simulink model "DCAC_conv_intconv_VSM"  (R2025a)
settings: Solver=VariableStepAuto  StartTime=0.0  StopTime=10.0  RelTol=1e-3
undefined symbols (not defined in the file): fb, Grid_op_VCVSC, Grid_op_VSM, Grid_opDC_VSM, Grid_opintconv_VSM, Grid_opVCVSC
libraries: simulink x1
(part 1 of 2)
settings Model: Creator=atomas  LastModifiedBy=atomas

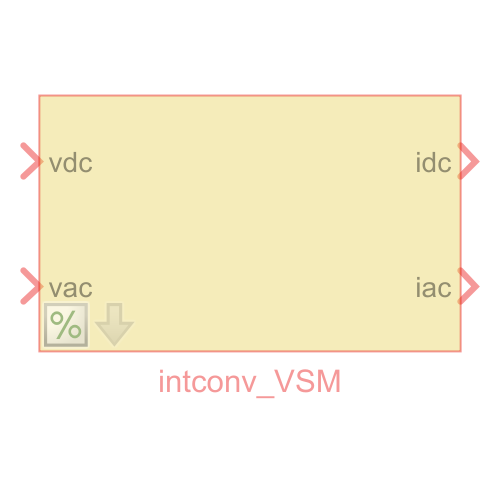
[thumbnail: Simulink's stored preview of the top-level diagram]
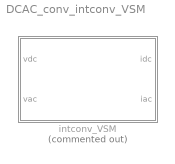
== system DCAC_conv_intconv_VSM ==
  intconv_VSM : Subsystem  Commented=on  mask(VCVSC){dynamic_VCC=Dynamic with P limitation, Lf=0.1, Rf=0.01, Rcf=1000000, Cfi=0.1, Kint=1, Tint=0.1, Bint=1, Kext=1, Bext=1, Text=0.1, Fi=1, Hv=3, Dv=0, Rv=0.05, nq=0.05, VI_L=0, VI_R=0, WOF_Tf=0, L_out=0.1, R_out=0.01}
      mask prompts: dynamic_VCC "Dynamic behavior"; Lf "Filter inductance (pu)"; Rf "Filter resistance (pu)"; Rcf "Parallel resistance to C (pu)"; Cfi "Filter capacitance (pu)"; Fi "Current feedfordward gain"; Hv "Inertia"; Dv "Damping"; Rv "Droop Rv"; nq "Droop nq"; VI_L "Inductance (pu)"; VI_R "Resistance (pu)"; WOF_Tf "WOF time constant (s)"; L_out "Output inductance (p.u.)"; R_out "Output resistance (p.u.)"
      mask help: Grid-forming converter. VCC are the voltage and current controllers. Dynamic behavior includes the PI controllers, decoupling, current feedfordward and LC output filter. Static behavior consists of setting the reference voltage directly in the output. PC is the power controller including the droop control and low-pass filters for the power measurements.
      mask init:
      | mdlWks = get_param(bdroot,'ModelWorkspace'); % Get the model workspace
      | block_name = get_param(gcb,'Name');
      | bvarname = get_param(get_param(get_param(...
      |         gcb, 'Parent'), 'Parent'), 'bvarname');
      | DC = mdlWks.getVariable([bvarname 'DC']);
      | try
      |     block_DC_buses = DC.(block_name + "s_DC_buses");
      |     block_buses = DC.(block_name + "s_buses");
      |     block_DC_toM = DC.(block_name + "s_DC_toM");
      |     block_toM = DC.(block_name + "s_toM");
      |     dparams = DC.(block_name + "_dparams");
      |     fref = mdlWks.getVariable([bvarname 'fref']);
      |     block_fref = fref.(block_name);
      | catch ME
      |     %errordlg(ME.message) 
      | end
      mask Help: web('Documentation/VCVSC.html')
      mask TypeOptions dynamic_VCC: Dynamic with limitation | Dynamic with P limitation | Dynamic | Static | Dynamic VC and static CC
      mask Callback dynamic_VCC:
      | block = gcb;
      | dynamic = get_param(block, 'dynamic_VCC');
      | param_vis = get_param(block,'MaskVisibilities');
      | block_params = string(fieldnames(get_param(block, 'DialogParameters')));
      | switch dynamic
      |     case 'Dynamic'
      |         param_vis(find(block_params == 'Lf'):find(block_params == 'Fi')) = cellstr("on");
      |         set_param([gcb '/VCC'], 'LabelModeActiveChoice', 'dynamic');
      |     case 'Dynamic with limitation'
      |         param_vis(find(block_params == 'Lf'):find(block_params == 'Fi')) = cellstr("on");
      |         set_param([gcb '/VCC'], 'LabelModeActiveChoice', 'dynamic_limiting');
      |     case 'Dynamic with P limitation'
      |         param_vis(find(block_params == 'Lf'):find(block_params == 'Fi')) = cellstr("on");
      |         set_param([gcb '/VCC'], 'LabelModeActiveChoice', 'dynamic_limiting_P');
      |     case 'Static'
      |         param_vis(find(block_params == 'Lf'):find(block_params == 'Fi')) = cellstr("off");
      |         set_param([gcb '/VCC'], 'LabelModeActiveChoice', 'static');
      |     case 'Dynamic VC and static CC'
      |         param_vis(find(block_params == 'Lf'):find(block_params == 'Fi')) = cellstr("on");
      |         param_vis(ismember(block_params, ["Lf","Rf","Kpc","Kic","Fi"])) = cellstr("off");
      |         set_param([gcb '/VCC'], 'LabelModeActiveChoice', 'dynamic_VC');
      | end
      | set_param(block,'MaskVisibilities',param_vis)
      mask TypeOptions VI_L: VI/L
      mask TypeOptions VI_R: VI/R
      mask TypeOptions WOF_Tf: VI/Tf
      mask DialogControl Container8 Prompt: Parameters
      mask DialogControl VCC Prompt: VCC
      mask DialogControl PC Prompt: PC
      mask DialogControl VI Prompt: VI
      mask DialogControl Container9 Prompt: Others

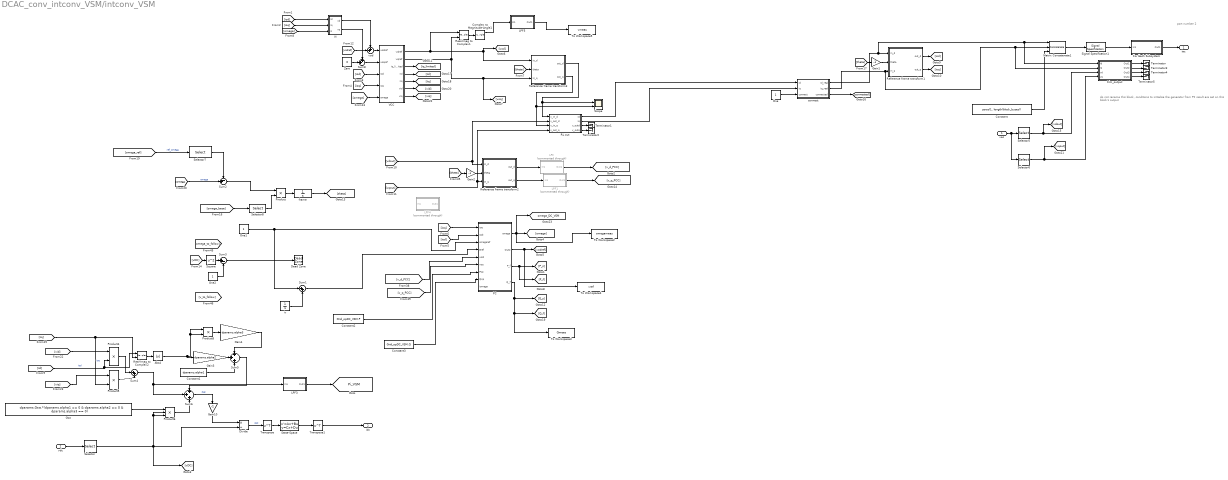
== system DCAC_conv_intconv_VSM/intconv_VSM ==
  note: port number 2
  note: do not rename this block, conditions to initialise the generator from PF result are set on this block's output
  vac : Inport
  vdc : Inport  Port=2
  Abs4 : Abs  SaturateOnIntegerOverflow=off
  Complex to Magnitude-Angle1 : ComplexToMagnitudeAngle
  Constant : Constant  Value=zeros(1, length(block_buses))  VectorParams1D=off
  Constant1 : Constant  Value=dparams.alpha1  VectorParams1D=off
  Constant2 : Constant  Value=Grid_opDC_VSM.P
  Constant3 : Constant  Value=Grid_opDC_VSM.Q
  Dead Zone : DeadZone  LowerValue=-0.2  UpperValue=0.2
  Divide : Product  Inputs=*/
  For Each Subsystem : Subsystem  TreatAsAtomicUnit=on
  Gain1 : Gain  Gain=-1
  Gain10 : Gain  Gain=-1
  Gain2 : Gain  Gain=-1
  Gain3 : Gain  Gain=dparams.alpha2
  Gain4 : Gain  Gain=dparams.alpha3
  Gsw : Constant  Value=dparams.Gsw.*(dparams.alpha1 == 0 & dparams.alpha2 == 0 & dparams.alpha3 == 0)  VectorParams1D=off
  LPF : Subsystem  Commented=through
  LPF1 : Subsystem  Commented=through
  LPF3 : Subsystem
  LPF4 : Subsystem  Commented=through
  LPF5 : Subsystem
  Matrix Concatenate1 : Concatenate  NumInputs=3  Mode=Multidimensional array
  One : Constant  OutDataTypeStr=Inherit: Inherit via back propagation
  One1 : Constant  OutDataTypeStr=Inherit: Inherit via back propagation
  One2 : Constant  OutDataTypeStr=Inherit: Inherit via back propagation
  PC : Subsystem  mask(PC_VCVSC){Tf=0.01, mp=0.01, nq=nq}
      mask prompts: Tf "Low-pass filter time constant (s)"; mp "Droop coefficient mp"; nq "Droop coefficient nq"
      mask help: Power controller of a grid-forming converter, including the droop control and low-pass filters for the power measurements.
      mask init:
      | if all(Tf ~= 0)
      |     iTf = 1./Tf;
      |     set_param([gcb '/LPF_P'],'Commented','off')
      |     set_param([gcb '/LPF_Q'],'Commented','off')
      | else
      |     set_param([gcb '/LPF_P'],'Commented','through')
      |     set_param([gcb '/LPF_Q'],'Commented','through')
      | end
  Product{,4..5,8} (4 alike) : Product
  Product6 : Product  Inputs=3
  RL out : Subsystem  Variant=on  VariantControlMode=label  LabelModeActiveChoice=dynamic  mask{dynamic=Dynamic, R=dparams.Rf, L=dparams.Lf, fbase=50}
      mask prompts: dynamic "Dynamic behavior"; R "Series resistance (p.u.)"; L "Inductance (p.u.)"; fbase "Base frequency (Hz)"
      mask init:
      | omegab = 2*pi*fbase;
      | invL = 1./L;
      | vssBlk = gcb;
      | switch dynamic
      |     case "Static"
      |         set_param(vssBlk, 'LabelModeActiveChoice', 'static');
      |     case "Dynamic"
      |         set_param(vssBlk, 'LabelModeActiveChoice', 'dynamic');
      |     case "Static omega"
      |         set_param(vssBlk, 'LabelModeActiveChoice', 'static_omega');
      | end
      mask TypeOptions dynamic: Static | Dynamic | Static omega
  Real-Imag to Complex1 : RealImagToComplex
  Real-Imag to Complex2 : RealImagToComplex
  Reference frame transform1 : Subsystem
  Reference frame transform2 : Subsystem
  Reference frame transform3 : Subsystem
  Scope : Scope  NumInputPorts=2
      settings: ActiveDisplayYMinimum=0.95813  ActiveDisplayYMaximum=1.0211
  Selector : Selector  InputPortWidth=DC.Nbuses  IndexOptions=Index vector (dialog)  Indices=block_DC_buses  OutputSizes=1
  Selector5 : Selector  NumberOfDimensions=2  InputPortWidth=3  IndexOptions=Index vector (dialog),Index vector (dialog)  Indices=1,block_buses  OutputSizes=1,1
  Selector6 : Selector  NumberOfDimensions=2  InputPortWidth=3  IndexOptions=Index vector (dialog),Index vector (dialog)  Indices=2,block_buses  OutputSizes=1,1
  Selector7 : Selector  InputPortWidth=length(fref.ref_units)  IndexOptions=Index vector (dialog)  Indices=block_fref  OutputSizes=1
  Selector8 : Selector  InputPortWidth=length(fref.ref_units)  IndexOptions=Index vector (dialog)  Indices=block_fref  OutputSizes=1
  Signal Specification1 : SignalSpecification  Dimensions=[3 length(block_buses)]
  Square : Math  Operator=square
  State-Space : StateSpace  A=[]  B=[]  C=[]  D=block_DC_toM  InitialCondition=0  ParameterTunability=Optimized
  Sum1 : Sum  Inputs=|++
  Sum2 : Sum  Inputs=-+|
  Sum3 : Sum  Inputs=|+-
  Sum4 : Sum  Inputs=|++
  Sum5 : Sum  Inputs=+|+|+
  Sum6 : Sum  Inputs=+|+|+
  Sum8 : Sum  Inputs=++|
  Terminator{,1..5} (6 alike) : Terminator
  To Workspace2 : ToWorkspace  VariableName=omegameas  SaveFormat=Timeseries  SampleTime=-1
  To Workspace3 : ToWorkspace  VariableName=Qmeas  SaveFormat=Timeseries  SampleTime=-1
  To Workspace4 : ToWorkspace  VariableName=vref  SaveFormat=Timeseries  SampleTime=-1
  To Workspace5 : ToWorkspace  VariableName=vmeas  SaveFormat=Timeseries  SampleTime=-1
  Transpose : Math  Operator=transpose
  Transpose1 : Math  Operator=transpose
  VCC : Subsystem  Variant=on  VariantControlMode=label  LabelModeActiveChoice=dynamic_limiting_P
  VI : Subsystem  mask{L=VI_L, R=VI_R, Tf=WOF_Tf}
      mask prompts: L "Inductance (pu)"; R "Resistance (pu)"; Tf "WOF time constant (s)"
      mask init:
      | if all(Tf ~= 0)
      |     iTf = 1./Tf;
      |     set_param([gcb '/WOF_d'],'Commented','off')
      |     set_param([gcb '/WOF_q'],'Commented','off')
      | else
      |     set_param([gcb '/WOF_d'],'Commented','through')
      |     set_param([gcb '/WOF_q'],'Commented','through')
      | end
  Zero : Constant  Value=0  OutDataTypeStr=Inherit: Inherit via back propagation
  connect : Subsystem
  frame : Integrator  InitialCondition=Grid_opintconv_VSM.frame  IgnoreLimit=on
  iv : Integrator  InitialCondition=Grid_opintconv_VSM.iv
  trim_output : Subsystem
  vod : Sum  Inputs=++|
  iac : Outport
  idc : Outport  Port=2
  tag scope: Pi_VSM=global, omega_DC_VSM=global
  wires:
  Selector7/1 -> Sum2/1
  Sum2/1 -> Product/1
  [omega_base] -> Selector8/1
  Selector8/1 -> Product/2
  LPF5/1(Out1) -> To Workspace5/1
  Complex to Magnitude-Angle1/1 -> LPF5/1(In1)
  Real-Imag to Complex1/1 -> Complex to Magnitude-Angle1/1
  LPF3/1(Out1) -> [Pi_VSM]
  Sum3/1 -> Dead Zone/1
  frame/1 -> [theta]
  One2/1 -> Sum3/2
  Square/1 -> Sum3/1
  [vDC] -> Square/1
  One1/1 -> Sum1/1, PC/3(omegaref)
  VCC/7(viq) -> [viq]
  VCC/6(vid) -> [vid]
  VCC/5(iiq) -> [iiq]
  VCC/4(iid) -> [iid]
  VCC/3(iq_limited) -> [iq_limited]
  Product/1 -> frame/1
  [iid] -> Real-Imag to Complex2/1, Product4/2  "iod"
  [vid] -> Product4/1
  [iiq] -> Real-Imag to Complex2/2, Product5/2  "ioq"
  Selector/1 -> Divide/2, [vDC], Product6/2, Product6/3
  [viq] -> Product5/1
  Product8/1 -> Gain4/1
  Gain10/1 -> Divide/1
  Gain3/1 -> Sum5/2
  Sum6/1 -> Gain10/1  "Pdc"
  Product4/1 -> Sum4/1
  Constant1/1 -> Sum5/3
  Real-Imag to Complex2/1 -> Abs4/1
  Gsw/1 -> Product6/1
  Gain4/1 -> Sum5/1
  State-Space/1 -> Transpose1/1
  Sum5/1 -> Sum6/1
  Sum4/1 -> Sum6/2, LPF3/1(In1)
  Product6/1 -> Sum6/3
  Product5/1 -> Sum4/2
  Transpose1/1 -> idc/1
  Abs4/1 -> Gain3/1, Product8/1, Product8/2
  Divide/1 -> Transpose/1  "iDC"
  Transpose/1 -> State-Space/1
  vdc/1 -> Selector/1
  Sum1/1 -> PC/4(Eref)
  One/1 -> connect/3(connect)
  iv/1 -> Sum1/2
  Constant3/1 -> PC/8(Qsp)
  Constant2/1 -> PC/7(Psp)
  VCC/2(viqref) -> Real-Imag to Complex1/2, Reference frame transform3/3(in_q), [voq]
  VCC/1(vidref) -> Reference frame transform3/1(in_d), [vod], Real-Imag to Complex1/1
  Selector5/1 -> trim_output/3(vd), [vdout]
  Selector6/1 -> trim_output/4(vq), [vqout]
  vac/1 -> Selector5/1, Selector6/1
  trim_output/4(Out4) -> Terminator5/1
  trim_output/3(Out3) -> Terminator4/1
  trim_output/2(Out2) -> Terminator3/1
  trim_output/1(Out1) -> Terminator/1
  [v_q_PCC] -> PC/6(voq)
  [v_d_PCC] -> PC/5(vodi)
  Signal Specification1/1 -> For Each Subsystem/1(In1)
  For Each Subsystem/1(Out1) -> iac/1
  Constant/1 -> Matrix Concatenate1/3
  Matrix Concatenate1/1 -> Signal Specification1/1
  [vdout] -> Reference frame transform2/1(in_d), RL out/2(v_out_d)
  LPF1/1(Out1) -> [v_q_PCC]
  LPF/1(Out1) -> [v_d_PCC]
  [vqout] -> RL out/4(v_out_q), Reference frame transform2/3(in_q)
  Reference frame transform2/2(out_q) -> LPF1/1(In1)
  Reference frame transform2/1(out_d) -> LPF/1(In1)
  RL out/4(v_outq) -> Terminator2/1
  RL out/3(v_outd) -> Terminator1/1
  connect/2(iq_real) -> Reference frame transform1/3(in_q), Matrix Concatenate1/2, trim_output/2(iq)
  connect/1(id_real) -> Reference frame transform1/1(in_d), Matrix Concatenate1/1, trim_output/1(id)
  VI/2(vq) -> Sum8/1
  VI/1(vd) -> vod/1
  Reference frame transform1/1(out_d) -> [iod]
  RL out/2(iq) -> connect/2(iq)
  Reference frame transform3/2(out_q) -> Scope/2, RL out/3(v_in_q)
  Reference frame transform3/1(out_d) -> Scope/1, RL out/1(v_in_d)
  Reference frame transform1/2(out_q) -> [ioq]
  [ioq] -> PC/1(ioq)
  [iod] -> PC/2(iodi)
  PC/2(Out2) -> [vodref], To Workspace4/1
  PC/1(omega) -> [omega], [omega_DC_VSM], To Workspace2/1
  [theta] -> Reference frame transform3/2(theta)
  [omega] -> VCC/5(omega)
  [vodref] -> vod/2
  Zero/1 -> Sum8/2
  [iod] -> VCC/3(iod)
  [ioq] -> VCC/4(ioq)
  Gain1/1 -> Reference frame transform1/2(theta)
  [theta] -> Gain1/1
  RL out/1(id) -> connect/1(id)
  [omega_ref] -> Selector7/1  "ref_omega"
  [omega] -> Sum2/2  "omega"
  connect/3(connected) -> [connected]
  PC/3(P_f) -> [P_f], [P_s]
  PC/4(Q_f) -> [Q_f], To Workspace3/1, [Q_s]
  [theta] -> Gain2/1
  Gain2/1 -> Reference frame transform2/2(theta)
  [iod] -> VI/1(id)
  [ioq] -> VI/2(iq)
  [omega] -> VI/3(omega)
  vod/1 -> VCC/1(vodref)
  Sum8/1 -> VCC/2(voqref)

== system DCAC_conv_intconv_VSM/intconv_VSM/For Each Subsystem ==
  In1 : Inport  Partition=on  PartitionDimension=1  PartitionWidth=1  PartitionOffset=0
  For Each : ForEach  DisableCoverage=on
  State-Space : StateSpace  A=[]  B=[]  C=[]  D=block_toM  InitialCondition=0  ParameterTunability=Optimized
  Transpose : Math  Operator=transpose
  Transpose1 : Math  Operator=transpose
  Out1 : Outport  ConcatenationDimension=1
  wires:
  In1/1 -> Transpose/1
  Transpose1/1 -> Out1/1
  Transpose/1 -> State-Space/1
  State-Space/1 -> Transpose1/1

== system DCAC_conv_intconv_VSM/intconv_VSM/LPF ==
  In1 : Inport
  Gain : Gain  Gain=1e2
  I : Integrator  InitialCondition=Grid_op_VCVSC.op.States(4).x'
  Sum4 : Sum  Inputs=|+-
  Out1 : Outport
  wires:
  I/1 -> Sum4/2, Out1/1
  In1/1 -> Sum4/1
  Sum4/1 -> Gain/1
  Gain/1 -> I/1

== system DCAC_conv_intconv_VSM/intconv_VSM/LPF1 ==
  In1 : Inport
  Gain : Gain  Gain=1e2
  I : Integrator  InitialCondition=Grid_op_VCVSC.op.States(5).x'
  Sum4 : Sum  Inputs=|+-
  Out1 : Outport
  wires:
  Gain/1 -> I/1
  Sum4/1 -> Gain/1
  In1/1 -> Sum4/1
  I/1 -> Out1/1, Sum4/2

== system DCAC_conv_intconv_VSM/intconv_VSM/LPF3 ==
  In1 : Inport
  Gain : Gain  Gain=1000
  I : Integrator
  Sum4 : Sum  Inputs=|+-
  Out1 : Outport
  wires:
  I/1 -> Sum4/2, Out1/1
  In1/1 -> Sum4/1
  Sum4/1 -> Gain/1
  Gain/1 -> I/1

== system DCAC_conv_intconv_VSM/intconv_VSM/LPF4 ==
  In1 : Inport
  Gain : Gain  Gain=1e2
  I : Integrator
  Sum4 : Sum  Inputs=|+-
  Out1 : Outport
  wires:
  I/1 -> Sum4/2, Out1/1
  In1/1 -> Sum4/1
  Sum4/1 -> Gain/1
  Gain/1 -> I/1

== system DCAC_conv_intconv_VSM/intconv_VSM/LPF5 ==
  In1 : Inport
  Gain : Gain  Gain=1e4
  I : Integrator  InitialConditionSource=external
  Sum4 : Sum  Inputs=|+-
  Out1 : Outport
  wires:
  I/1 -> Sum4/2, Out1/1
  In1/1 -> Sum4/1, I/2
  Sum4/1 -> Gain/1
  Gain/1 -> I/1

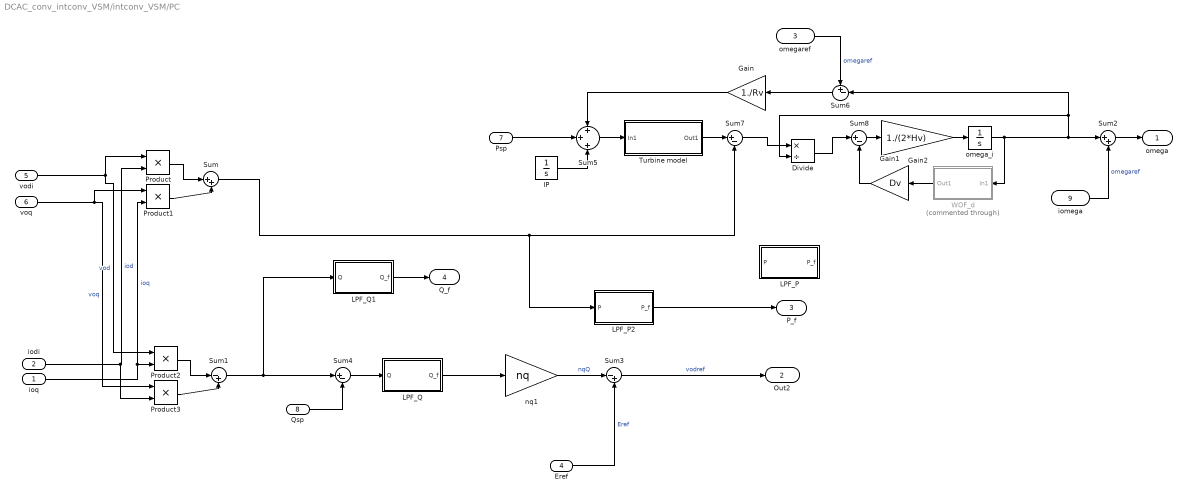
== system DCAC_conv_intconv_VSM/intconv_VSM/PC ==
  ioq : Inport
  iodi : Inport  Port=2
  omegaref : Inport  Port=3
  Eref : Inport  Port=4
  vodi : Inport  Port=5
  voq : Inport  Port=6
  Psp : Inport  Port=7
  Qsp : Inport  Port=8
  iomega : Inport  Port=9
  Divide : Product  Inputs=*/
  Gain : Gain  Gain=1./Rv
  Gain1 : Gain  Gain=Dv
  Gain2 : Gain  Gain=1./(2*Hv)
  IP : Integrator  InitialCondition=Grid_opintconv_VSM.IP
  LPF_P : Subsystem
  LPF_P2 : Subsystem
  LPF_Q : Subsystem
  LPF_Q1 : Subsystem
  Product{,1..3} (4 alike) : Product
  Sum : Sum  Inputs=|++
  Sum1 : Sum  Inputs=|-+
  Sum2 : Sum  Inputs=|++
  Sum3 : Sum  Inputs=|-+
  Sum4 : Sum  Inputs=|+-
  Sum5 : Sum  Inputs=+|+|+
  Sum6 : Sum  Inputs=+-|
  Sum7 : Sum  Inputs=|+-
  Sum8 : Sum  Inputs=|+-
  Turbine model : Subsystem
  WOF_d : Subsystem  Commented=through
  nq1 : Gain  Gain=nq
  omega_i : Integrator  InitialCondition=1
  omega : Outport
  Out2 : Outport  Port=2
  P_f : Outport  Port=3
  Q_f : Outport  Port=4
  wires:
  LPF_Q1/1(Q_f) -> Q_f/1
  LPF_P2/1(P_f) -> P_f/1
  iomega/1 -> Sum2/2  "omegaref"
  Sum2/1 -> omega/1
  omegaref/1 -> Sum6/1  "omegaref"
  IP/1 -> Sum5/3
  Sum8/1 -> Gain2/1
  Sum7/1 -> Divide/1
  Sum5/1 -> Turbine model/1(In1)
  Psp/1 -> Sum5/2
  Divide/1 -> Sum8/1
  Gain1/1 -> Sum8/2
  Turbine model/1(Out1) -> Sum7/1
  WOF_d/1(Out1) -> Gain1/1
  Gain/1 -> Sum5/1
  omega_i/1 -> Divide/2, Sum6/2, Sum2/1, WOF_d/1(In1)
  Sum/1 -> LPF_P2/1(P), Sum7/2
  Sum6/1 -> Gain/1
  Gain2/1 -> omega_i/1
  LPF_Q/1(Q_f) -> nq1/1
  Sum3/1 -> Out2/1  "vodref"
  Sum4/1 -> LPF_Q/1(Q)
  Qsp/1 -> Sum4/2
  ioq/1 -> Product1/2, Product2/2  "ioq"
  iodi/1 -> Product/2, Product3/2  "iod"
  voq/1 -> Product3/1, Product1/1  "voq"
  Sum1/1 -> Sum4/1, LPF_Q1/1(Q)
  Eref/1 -> Sum3/2  "Eref"
  nq1/1 -> Sum3/1  "nqQ"
  Product3/1 -> Sum1/2
  Product2/1 -> Sum1/1
  Product1/1 -> Sum/2
  Product/1 -> Sum/1
  vodi/1 -> Product/1, Product2/1  "vod"

== system DCAC_conv_intconv_VSM/intconv_VSM/RL out ==
  note: 1) Add Subsystem or Model blocks as valid variant choices.
      | 2) You cannot connect blocks at this level. At simulation, connectivity is automatically
      | determined, based on the active variant and port name matching.
  v_in_d : Inport
  v_out_d : Inport  Port=2
  v_in_q : Inport  Port=3
  v_out_q : Inport  Port=4
  dynamic : Subsystem  VariantControl=dynamic
  static : Subsystem  VariantControl=static
  static_omega : Subsystem  VariantControl=static_omega
  id : Outport
  iq : Outport  Port=2
  v_outd : Outport  Port=3
  v_outq : Outport  Port=4

== system DCAC_conv_intconv_VSM/intconv_VSM/Reference frame transform1 ==
  in_d : Inport
  theta : Inport  Port=2
  in_q : Inport  Port=3
  Complex to Real-Imag : ComplexToRealImag
  Cos : Trigonometry  SCDEnableBlockLinearizationSpecification=on  Operator=cos
  Product : Product
  Real-Imag to Complex : RealImagToComplex
  Real-Imag to Complex1 : RealImagToComplex
  Sin : Trigonometry  SCDEnableBlockLinearizationSpecification=on
  out_d : Outport
  out_q : Outport  Port=2
  wires:
  in_d/1 -> Real-Imag to Complex/1
  in_q/1 -> Real-Imag to Complex/2
  Complex to Real-Imag/1 -> out_d/1
  Sin/1 -> Real-Imag to Complex1/2
  Cos/1 -> Real-Imag to Complex1/1
  theta/1 -> Cos/1, Sin/1
  Product/1 -> Complex to Real-Imag/1
  Real-Imag to Complex/1 -> Product/2
  Real-Imag to Complex1/1 -> Product/1
  Complex to Real-Imag/2 -> out_q/1

== system DCAC_conv_intconv_VSM/intconv_VSM/Reference frame transform2 ==
  in_d : Inport
  theta : Inport  Port=2
  in_q : Inport  Port=3
  Complex to Real-Imag : ComplexToRealImag
  Cos : Trigonometry  SCDEnableBlockLinearizationSpecification=on  Operator=cos
  Product : Product
  Real-Imag to Complex : RealImagToComplex
  Real-Imag to Complex1 : RealImagToComplex
  Sin : Trigonometry  SCDEnableBlockLinearizationSpecification=on
  out_d : Outport
  out_q : Outport  Port=2
  wires:
  Complex to Real-Imag/2 -> out_q/1
  Real-Imag to Complex1/1 -> Product/1
  Real-Imag to Complex/1 -> Product/2
  Product/1 -> Complex to Real-Imag/1
  theta/1 -> Sin/1, Cos/1
  Cos/1 -> Real-Imag to Complex1/1
  Sin/1 -> Real-Imag to Complex1/2
  Complex to Real-Imag/1 -> out_d/1
  in_q/1 -> Real-Imag to Complex/2
  in_d/1 -> Real-Imag to Complex/1

== system DCAC_conv_intconv_VSM/intconv_VSM/Reference frame transform3 ==
  in_d : Inport
  theta : Inport  Port=2
  in_q : Inport  Port=3
  Complex to Real-Imag : ComplexToRealImag
  Cos : Trigonometry  SCDEnableBlockLinearizationSpecification=on  Operator=cos
  Product : Product
  Real-Imag to Complex : RealImagToComplex
  Real-Imag to Complex1 : RealImagToComplex
  Sin : Trigonometry  SCDEnableBlockLinearizationSpecification=on
  out_d : Outport
  out_q : Outport  Port=2
  wires:
  in_d/1 -> Real-Imag to Complex/1
  in_q/1 -> Real-Imag to Complex/2
  Complex to Real-Imag/1 -> out_d/1
  Sin/1 -> Real-Imag to Complex1/2
  Cos/1 -> Real-Imag to Complex1/1
  theta/1 -> Sin/1, Cos/1
  Product/1 -> Complex to Real-Imag/1
  Real-Imag to Complex/1 -> Product/2
  Real-Imag to Complex1/1 -> Product/1
  Complex to Real-Imag/2 -> out_q/1

== system DCAC_conv_intconv_VSM/intconv_VSM/VCC ==
  note: 1) Add Subsystem or Model blocks as valid variant choices.
      | 2) You cannot connect blocks at this level. At simulation, connectivity is automatically
      | determined, based on the active variant and port name matching.
  vodref : Inport
  voqref : Inport  Port=2
  iod : Inport  Port=3
  ioq : Inport  Port=4
  omega : Inport  Port=5
  dynamic : Subsystem  VariantControl=dynamic
  dynamic_VC : Subsystem  VariantControl=dynamic_VC
  dynamic_limiting : Subsystem  VariantControl=dynamic_limiting
  dynamic_limiting_P : Subsystem  VariantControl=dynamic_limiting_P
  static : Subsystem  VariantControl=static
  vidref : Outport
  viqref : Outport  Port=2
  iq_limited : Outport  Port=3
  iid : Outport  Port=4
  iiq : Outport  Port=5
  vid : Outport  Port=6
  viq : Outport  Port=7

== system DCAC_conv_intconv_VSM/intconv_VSM/VI ==
  id : Inport
  iq : Inport  Port=2
  omega : Inport  Port=3
  Gain : Gain  Gain=L
  Gain1 : Gain  Gain=R
  Gain2 : Gain  Gain=L
  Gain3 : Gain  Gain=R
  Product : Product
  Product1 : Product
  Sum : Sum  Inputs=-+|
  Sum1 : Sum  Inputs=|--
  WOF_d : Subsystem  Commented=through
  WOF_q : Subsystem  Commented=through
  vd : Outport
  vq : Outport  Port=2
  wires:
  Gain/1 -> Product/1
  omega/1 -> Product/2, Product1/1
  iq/1 -> WOF_q/1(In1)
  Product/1 -> Sum/2
  id/1 -> WOF_d/1(In1)
  Gain2/1 -> Product1/2
  Product1/1 -> Sum1/1
  Gain1/1 -> Sum/1
  Gain3/1 -> Sum1/2
  Sum/1 -> vd/1
  Sum1/1 -> vq/1
  WOF_d/1(Out1) -> Gain2/1, Gain1/1
  WOF_q/1(Out1) -> Gain3/1, Gain/1

== system DCAC_conv_intconv_VSM/intconv_VSM/connect ==
  id : Inport
  iq : Inport  Port=2
  connect : Inport  Port=3
  Switch : Switch  Criteria=u2 > Threshold  ZeroCross=off  SaturateOnIntegerOverflow=off  InputSameDT=off
  Switch1 : Switch  Criteria=u2 > Threshold  ZeroCross=off  SaturateOnIntegerOverflow=off  InputSameDT=off
  Zero1 : Constant  Value=0  VectorParams1D=off  OutDataTypeStr=Inherit: Inherit via back propagation
  Zero2 : Constant  Value=0  VectorParams1D=off  OutDataTypeStr=Inherit: Inherit via back propagation
  id_real : Outport
  iq_real : Outport  Port=2
  connected : Outport  Port=3  OutDataTypeStr=boolean
  wires:
  Zero2/1 -> Switch1/3
  iq/1 -> Switch1/1
  Switch1/1 -> iq_real/1
  connect/1 -> Switch/2, Switch1/2, connected/1
  id/1 -> Switch/1
  Zero1/1 -> Switch/3
  Switch/1 -> id_real/1

== system DCAC_conv_intconv_VSM/intconv_VSM/trim_output ==
  id : Inport
  iq : Inport  Port=2
  vd : Inport  Port=3
  vq : Inport  Port=4
  Out1 : Outport
  Out2 : Outport  Port=2
  Out3 : Outport  Port=3
  Out4 : Outport  Port=4
  wires:
  iq/1 -> Out2/1
  vd/1 -> Out3/1
  vq/1 -> Out4/1
  id/1 -> Out1/1

== system DCAC_conv_intconv_VSM/intconv_VSM/PC/LPF_P ==
  P : Inport
  Gain : Gain  Gain=1e4
  I : Integrator  InitialCondition=Grid_opintconv_VSM.P
  Sum4 : Sum  Inputs=|+-
  P_f : Outport
  wires:
  I/1 -> Sum4/2, P_f/1
  P/1 -> Sum4/1
  Sum4/1 -> Gain/1
  Gain/1 -> I/1

== system DCAC_conv_intconv_VSM/intconv_VSM/PC/LPF_P2 ==
  P : Inport
  Gain : Gain  Gain=1e4
  I : Integrator  InitialCondition=Grid_opDC_VSM.P
  Sum4 : Sum  Inputs=|+-
  P_f : Outport
  wires:
  Gain/1 -> I/1
  Sum4/1 -> Gain/1
  P/1 -> Sum4/1
  I/1 -> P_f/1, Sum4/2

== system DCAC_conv_intconv_VSM/intconv_VSM/PC/LPF_Q ==
  Q : Inport
  Gain : Gain  Gain=iTf
  I : Integrator
  Sum4 : Sum  Inputs=|+-
  Q_f : Outport
  wires:
  Sum4/1 -> Gain/1
  I/1 -> Sum4/2, Q_f/1
  Q/1 -> Sum4/1
  Gain/1 -> I/1

== system DCAC_conv_intconv_VSM/intconv_VSM/PC/LPF_Q1 ==
  Q : Inport
  Gain : Gain  Gain=iTf
  I : Integrator  InitialConditionSource=external
  Sum4 : Sum  Inputs=|+-
  Q_f : Outport
  wires:
  Gain/1 -> I/1
  Q/1 -> Sum4/1, I/2
  I/1 -> Q_f/1, Sum4/2
  Sum4/1 -> Gain/1

== system DCAC_conv_intconv_VSM/intconv_VSM/PC/Turbine model ==
  In1 : Inport
  Out1 : Outport
  wires:
  In1/1 -> Out1/1

== system DCAC_conv_intconv_VSM/intconv_VSM/PC/WOF_d ==
  In1 : Inport
  Gain : Gain  Gain=10
  Gain1 : Gain  Gain=10
  I : Integrator  InitialConditionSource=external  InitialCondition=Grid_op_VSM.op.States(7).x'
  Sum : Sum  Inputs=+-|
  Sum4 : Sum  Inputs=|+-
  Out1 : Outport
  wires:
  Gain1/1 -> Out1/1
  Sum/1 -> Gain1/1
  I/1 -> Sum4/2, Sum/2
  In1/1 -> Sum4/1, Sum/1, I/2
  Sum4/1 -> Gain/1
  Gain/1 -> I/1

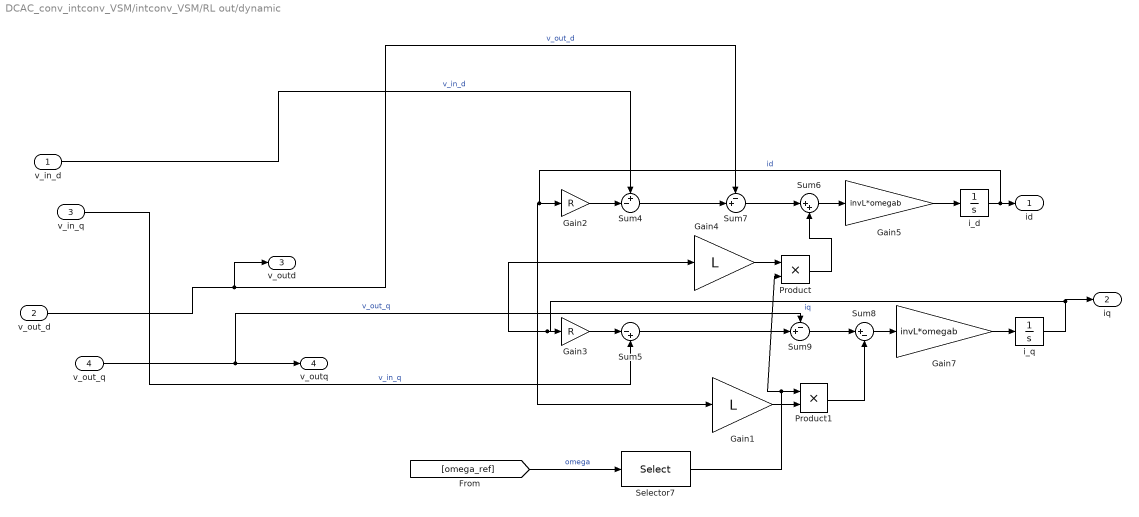
== system DCAC_conv_intconv_VSM/intconv_VSM/RL out/dynamic ==
  v_in_d : Inport
  v_out_d : Inport  Port=2
  v_in_q : Inport  Port=3
  v_out_q : Inport  Port=4
  Gain1 : Gain  Gain=L
  Gain2 : Gain  Gain=R
  Gain3 : Gain  Gain=R
  Gain4 : Gain  Gain=L
  Gain5 : Gain  Gain=invL*omegab
  Gain7 : Gain  Gain=invL*omegab
  Product : Product
  Product1 : Product
  Selector7 : Selector  InputPortWidth=length(fref.ref_units)  IndexOptions=Index vector (dialog)  Indices=block_fref  OutputSizes=1
  Sum4 : Sum  Inputs=+-|
  Sum5 : Sum  Inputs=|-+
  Sum6 : Sum  Inputs=|++
  Sum7 : Sum  Inputs=-+|
  Sum8 : Sum  Inputs=|+-
  Sum9 : Sum  Inputs=-+|
  i_d : Integrator  InitialCondition=Grid_opintconv_VSM.id_out
  i_q : Integrator  InitialCondition=Grid_opintconv_VSM.iq_out
  id : Outport
  iq : Outport  Port=2
  v_outd : Outport  Port=3
  v_outq : Outport  Port=4
  wires:
  Selector7/1 -> Product1/1, Product/2
  v_in_q/1 -> Sum5/2  "v_in_q"
  v_in_d/1 -> Sum4/1  "v_in_d"
  Gain2/1 -> Sum4/2
  i_d/1 -> Gain2/1, Gain1/1, id/1  "id"
  Sum6/1 -> Gain5/1
  [omega_ref] -> Selector7/1  "omega"
  Gain5/1 -> i_d/1
  Product/1 -> Sum6/2
  Sum8/1 -> Gain7/1
  Sum4/1 -> Sum7/2
  Product1/1 -> Sum8/2
  Gain4/1 -> Product/1
  Sum7/1 -> Sum6/1
  Gain3/1 -> Sum5/1
  Sum5/1 -> Sum9/2
  Gain7/1 -> i_q/1
  i_q/1 -> Gain3/1, Gain4/1, iq/1  "iq"
  Gain1/1 -> Product1/2
  Sum9/1 -> Sum8/1
  v_out_d/1 -> Sum7/1, v_outd/1  "v_out_d"
  v_out_q/1 -> Sum9/1, v_outq/1  "v_out_q"

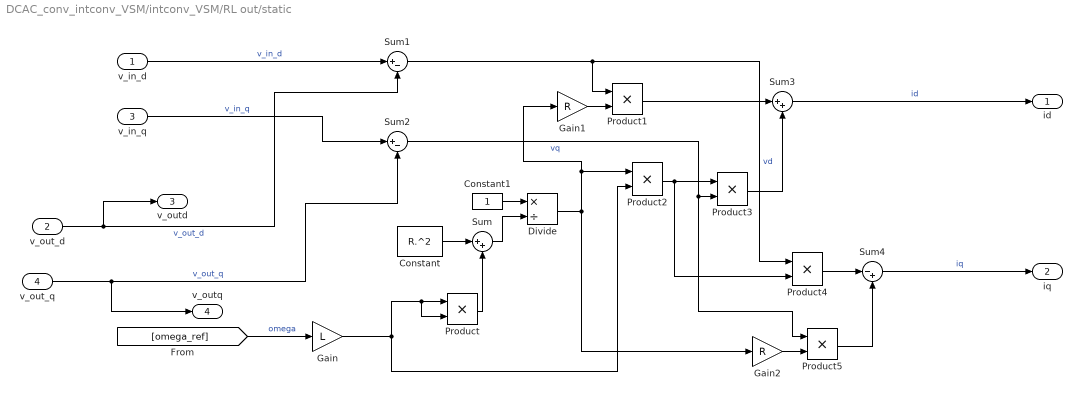
== system DCAC_conv_intconv_VSM/intconv_VSM/RL out/static ==
  v_in_d : Inport
  v_out_d : Inport  Port=2
  v_in_q : Inport  Port=3
  v_out_q : Inport  Port=4
  Constant : Constant  Value=R.^2
  Constant1 : Constant
  Divide : Product  Inputs=*/
  Gain : Gain  Gain=L
  Gain1 : Gain  Gain=R
  Gain2 : Gain  Gain=R
  Product{,1..5} (6 alike) : Product
  Sum : Sum  Inputs=|++
  Sum1 : Sum  Inputs=|+-
  Sum2 : Sum  Inputs=|+-
  Sum3 : Sum  Inputs=|++
  Sum4 : Sum  Inputs=|-+
  id : Outport
  iq : Outport  Port=2
  v_outd : Outport  Port=3
  v_outq : Outport  Port=4
  wires:
  v_in_q/1 -> Sum2/1  "v_in_q"
  v_out_d/1 -> Sum1/2, v_outd/1  "v_out_d"
  Sum/1 -> Divide/2
  Gain2/1 -> Product5/2
  Product/1 -> Sum/2
  Product1/1 -> Sum3/1
  Product5/1 -> Sum4/2
  Constant/1 -> Sum/1
  Sum2/1 -> Product3/2, Product5/1  "vq"
  Gain/1 -> Product2/2, Product/1, Product/2
  Constant1/1 -> Divide/1
  Product3/1 -> Sum3/2
  Sum1/1 -> Product4/1, Product1/1  "vd"
  Divide/1 -> Product2/1, Gain1/1, Gain2/1
  Product4/1 -> Sum4/1
  Product2/1 -> Product3/1, Product4/2
  Gain1/1 -> Product1/2
  Sum3/1 -> id/1  "id"
  Sum4/1 -> iq/1  "iq"
  v_out_q/1 -> Sum2/2, v_outq/1  "v_out_q"
  v_in_d/1 -> Sum1/1  "v_in_d"
  [omega_ref] -> Gain/1  "omega"

== system DCAC_conv_intconv_VSM/intconv_VSM/RL out/static_omega ==
  v_in_d : Inport
  v_out_d : Inport  Port=2
  v_in_q : Inport  Port=3
  v_out_q : Inport  Port=4
  Gain : Gain  Gain=1./(R.^2+L.^2)
  Gain2 : Gain  Gain=1./(R.^2+L.^2)
  Gain3 : Gain  Gain=R
  Gain4 : Gain  Gain=L
  Gain5 : Gain  Gain=L
  Gain6 : Gain  Gain=R
  Sum : Sum  Inputs=|++
  Sum1 : Sum  Inputs=|+-
  Sum2 : Sum  Inputs=|+-
  Sum3 : Sum  Inputs=|-+
  id : Outport
  iq : Outport  Port=2
  v_outd : Outport  Port=3
  v_outq : Outport  Port=4
  wires:
  Gain6/1 -> Sum3/2
  Sum3/1 -> iq/1
  Gain5/1 -> Sum3/1
  Sum/1 -> id/1
  Gain2/1 -> Gain4/1, Gain6/1
  Gain4/1 -> Sum/2
  Gain3/1 -> Sum/1
  Gain/1 -> Gain3/1, Gain5/1
  Sum2/1 -> Gain2/1  "vq"
  Sum1/1 -> Gain/1  "vd"
  v_out_d/1 -> Sum1/2, v_outd/1  "v_out_d"
  v_out_q/1 -> Sum2/2, v_outq/1  "v_out_q"
  v_in_d/1 -> Sum1/1  "v_in_d"
  v_in_q/1 -> Sum2/1  "v_in_q"

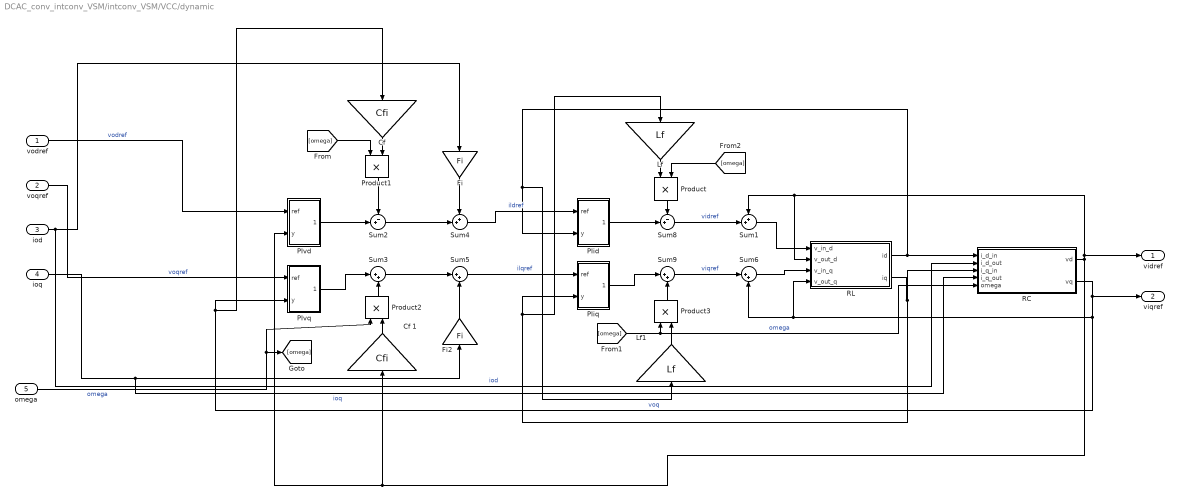
== system DCAC_conv_intconv_VSM/intconv_VSM/VCC/dynamic ==
  vodref : Inport
  voqref : Inport  Port=2
  iod : Inport  Port=3
  ioq : Inport  Port=4
  omega : Inport  Port=5
  Cf : Gain  Gain=Cfi
  Cf 1 : Gain  Gain=Cfi
  Fi : Gain  Gain=Fi
  Fi2 : Gain  Gain=Fi
  "Lf " : Gain  Gain=Lf
  Lf1 : Gain  Gain=Lf
  PIid : Subsystem
  PIiq : Subsystem
  PIvd : Subsystem
  PIvq : Subsystem
  Product{,1..3} (4 alike) : Product
  RC : Subsystem  Variant=on  VariantControlMode=label  LabelModeActiveChoice=dynamic  mask{dynamic=Dynamic, R=Rcf, C=Cfi, fbase=50}
      mask prompts: dynamic "Dynamic behavior"; R "Parallel resistance (p.u.)"; C "Capacitance (p.u.)"; fbase "Base frequency (Hz)"
      mask init:
      | omegab = 2*pi*fbase;
      | iC = 1./C;
      | iR = 1./R;
      | vssBlk = gcb;
      | switch dynamic
      |     case "Dynamic"
      |         set_param(vssBlk, 'LabelModeActiveChoice', 'dynamic');
      |     case "Static"
      |         set_param(vssBlk, 'LabelModeActiveChoice', 'static');
      |     case "Static omega"
      |         set_param(vssBlk, 'LabelModeActiveChoice', 'static omega');
      | end
      mask TypeOptions dynamic: Dynamic | Static | Static omega
  RL : Subsystem  Variant=on  VariantControlMode=label  LabelModeActiveChoice=dynamic  mask(Line){dynamic=Dynamic, R=Rf, L=Lf, fbase=fb}
      mask prompts: dynamic "Dynamic behavior"; R "Series resistance (p.u.)"; L "Inductance (p.u.)"; fbase "Base frequency (Hz)"
      mask init: same as DCAC_conv_intconv_VSM/intconv_VSM/RL out
      mask Help: web('Documentation/RL.html')
      mask TypeOptions dynamic: Static | Dynamic | Static omega
  Sum1 : Sum  Inputs=++|
  Sum2 : Sum  Inputs=-+|
  Sum{3,5..6,9} (4 alike) : Sum  Inputs=|++
  Sum4 : Sum  Inputs=++|
  Sum8 : Sum  Inputs=-+|
  vidref : Outport
  viqref : Outport  Port=2
  wires:
  Sum6/1 -> RL/3(v_in_q)
  Sum1/1 -> RL/1(v_in_d)
  Sum9/1 -> Sum6/1  "viqref"
  Sum8/1 -> Sum1/2  "vidref"
  RL/2(iq) -> "Lf "/1, PIiq/2(y), RC/3(i_q_in)
  RL/1(id) -> RC/1(i_d_in), Lf1/1, PIid/2(y)
  RC/1(vd) -> Cf 1/1, PIvd/2(y), RL/2(v_out_d), Sum1/1, vidref/1
  [omega] -> Product1/1
  omega/1 -> [omega], Product2/1  "omega"
  PIiq/1(Out1) -> Sum9/1
  PIid/1(Out1) -> Sum8/2
  PIvq/1(Out1) -> Sum3/1
  PIvd/1(Out1) -> Sum2/2
  Fi2/1 -> Sum5/2
  ioq/1 -> Fi2/1, RC/4(i_q_out)  "ioq"
  [omega] -> Product3/1, RC/5(omega)  "omega"
  Sum3/1 -> Sum5/1
  "Lf "/1 -> Product/1
  Sum2/1 -> Sum4/2
  iod/1 -> Fi/1, RC/2(i_d_out)  "iod"
  Product1/1 -> Sum2/1
  Sum4/1 -> PIid/1(ref)  "ildref"
  Cf/1 -> Product1/2
  Cf 1/1 -> Product2/2
  Product2/1 -> Sum3/2
  Product3/1 -> Sum9/2
  voqref/1 -> PIvq/1(ref)  "voqref"
  Fi/1 -> Sum4/1
  Lf1/1 -> Product3/2
  [omega] -> Product/2
  RC/2(vq) -> Cf/1, PIvq/2(y), RL/4(v_out_q), Sum6/2, viqref/1  "voq"
  vodref/1 -> PIvd/1(ref)  "vodref"
  Product/1 -> Sum8/1
  Sum5/1 -> PIiq/1(ref)  "ilqref"

== system DCAC_conv_intconv_VSM/intconv_VSM/VCC/dynamic_VC ==
  vodref : Inport
  voqref : Inport  Port=2
  iod : Inport  Port=3
  ioq : Inport  Port=4
  omega : Inport  Port=5
  Cf : Gain  Gain=Cfi
  Cf 1 : Gain  Gain=Cfi
  Fi : Gain  Gain=Fi
  Fi2 : Gain  Gain=Fi
  Product1 : Product
  Product2 : Product
  RC : Subsystem  Variant=on  VariantControlMode=label  LabelModeActiveChoice=dynamic  mask{dynamic=Dynamic, R=Rcf, C=Cfi, fbase=50}
      mask prompts: dynamic "Dynamic behavior"; R "Parallel resistance (p.u.)"; C "Capacitance (p.u.)"; fbase "Base frequency (Hz)"
      mask init: same as DCAC_conv_intconv_VSM/intconv_VSM/VCC/dynamic/RC
      mask TypeOptions dynamic: Dynamic | Static | Static omega
  Subsystem : Subsystem
  Subsystem1 : Subsystem
  Sum2 : Sum  Inputs=-+|
  Sum3 : Sum  Inputs=|++
  Sum4 : Sum  Inputs=++|
  Sum5 : Sum  Inputs=|++
  vidref : Outport
  viqref : Outport  Port=2
  wires:
  Sum5/1 -> RC/3(i_q_in)
  Sum4/1 -> RC/1(i_d_in)
  RC/1(v_d) -> Subsystem/2(y), Cf 1/1, vidref/1
  vodref/1 -> Subsystem/1(ref)  "vodref"
  RC/2(v_q) -> Subsystem1/2(y), Cf/1, viqref/1
  Fi/1 -> Sum4/1
  voqref/1 -> Subsystem1/1(ref)  "voqref"
  Product2/1 -> Sum3/2
  Cf 1/1 -> Product2/2
  Cf/1 -> Product1/2
  Product1/1 -> Sum2/1
  iod/1 -> Fi/1, RC/2(i_d_out)  "iod"
  Sum2/1 -> Sum4/2
  Sum3/1 -> Sum5/1
  ioq/1 -> Fi2/1, RC/4(i_q_out)  "ioq"
  Fi2/1 -> Sum5/2
  Subsystem/1(Out1) -> Sum2/2
  Subsystem1/1(Out1) -> Sum3/1
  omega/1 -> [omega], Product2/1, RC/5(omega)  "omega"
  [omega] -> Product1/1

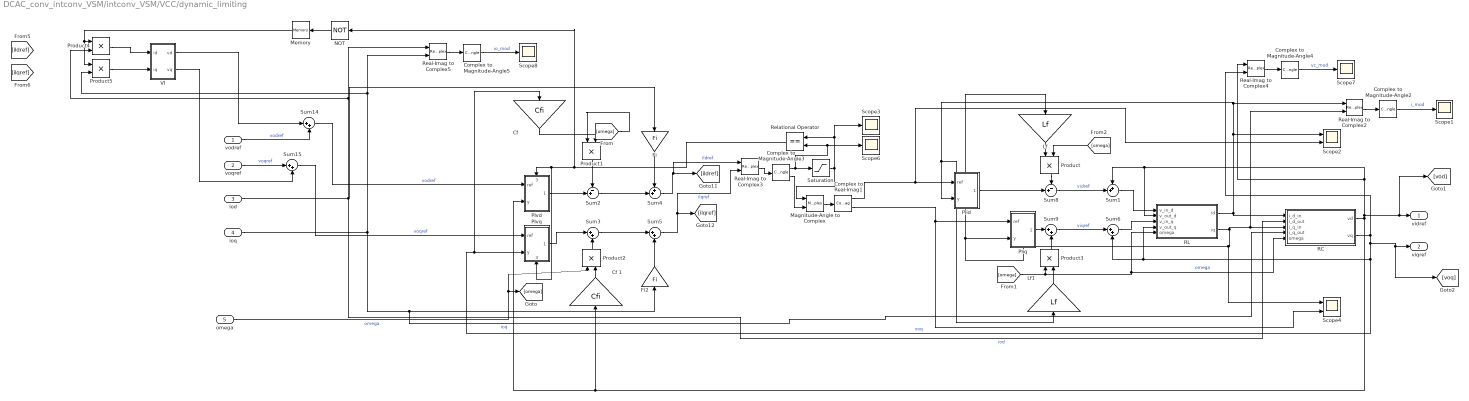
== system DCAC_conv_intconv_VSM/intconv_VSM/VCC/dynamic_limiting ==
  vodref : Inport
  voqref : Inport  Port=2
  iod : Inport  Port=3
  ioq : Inport  Port=4
  omega : Inport  Port=5
  Cf : Gain  Gain=Cfi
  Cf 1 : Gain  Gain=Cfi
  Complex to Magnitude-Angle2 : ComplexToMagnitudeAngle  Output=Magnitude
  Complex to Magnitude-Angle3 : ComplexToMagnitudeAngle
  Complex to Magnitude-Angle4 : ComplexToMagnitudeAngle  Output=Magnitude
  Complex to Magnitude-Angle5 : ComplexToMagnitudeAngle  Output=Magnitude
  Complex to Real-Imag1 : ComplexToRealImag
  Fi : Gain  Gain=Fi
  Fi2 : Gain  Gain=Fi
  "Lf " : Gain  Gain=Lf
  Lf1 : Gain  Gain=Lf
  Magnitude-Angle to Complex : MagnitudeAngleToComplex
  Memory : Memory
  NOT : Logic  Operator=NOT  IconShape=distinctive  AllPortsSameDT=off  OutDataTypeStr=boolean
  PIid : Subsystem
  PIiq : Subsystem
  PIvd : Subsystem
      settings: PortSchema="{\"entries\":[{\"content\":{\"sides\":[{\"content\":{\"connectorIds\":[\"In1\",\"In2\"]},\"type\":\"ConnectorPlacement.EquallySpacedRectSide\",\"uuid\":\"218efe14-094c-4cdd-8e62-ef6089c75bbd\"},{\"content\":{\"connectorIds\":[\"Out1\"],\"side\":\"RIGHT\"},\"type\":\"ConnectorPlacement.EquallySpacedRectSide\",\"uuid\":\"287e2a8a-062a-4519-a86c-f141c6982dac\"},{\"content\":{\"connectorIds\":[\"In3\"],\"side\":\"TOP\"},\"type\":\"ConnectorPlacement.EquallySpacedRectSide\",\"uuid\":\"e88fce21-908c-492a-b265-04b05ce94be8\"}]},\"type\":\"ConnectorPlacement.EquallySpacedConnector\",\"uuid\":\"5c149457-da6d-4223-b1cb-56365173b759\"}],\"packageUris\":[\"http://schema.mathworks.com/mf0/Connector/R2020b\"],\"version\":\"1.0\"}"
  PIvq : Subsystem
      settings: PortSchema="{\"entries\":[{\"content\":{\"sides\":[{\"content\":{\"connectorIds\":[\"In1\",\"In2\"]},\"type\":\"ConnectorPlacement.EquallySpacedRectSide\",\"uuid\":\"218efe14-094c-4cdd-8e62-ef6089c75bbd\"},{\"content\":{\"connectorIds\":[\"Out1\"],\"side\":\"RIGHT\"},\"type\":\"ConnectorPlacement.EquallySpacedRectSide\",\"uuid\":\"287e2a8a-062a-4519-a86c-f141c6982dac\"},{\"content\":{\"connectorIds\":[],\"side\":\"TOP\"},\"type\":\"ConnectorPlacement.EquallySpacedRectSide\",\"uuid\":\"e88fce21-908c-492a-b265-04b05ce94be8\"},{\"content\":{\"connectorIds\":[\"In3\"],\"side\":\"BOTTOM\"},\"type\":\"ConnectorPlacement.EquallySpacedRectSide\",\"uuid\":\"db964aea-37c6-4226-90b6-d177a6d2ab38\"}]},\"type\":\"ConnectorPlacement.EquallySpacedConnector\",\"uuid\":\"5c149457-da6d-4223-b1cb-56365173b759\"}],\"packageUris\":[\"http://schema.mathworks.com/mf0/Connector/R2020b\"],\"version\":\"1.0\"}"
  Product{,1..5} (6 alike) : Product
  RC : Subsystem  Variant=on  VariantControlMode=label  LabelModeActiveChoice=dynamic  mask{dynamic=Dynamic, R=Rcf, C=Cfi}
      mask prompts: dynamic "Dynamic behavior"; R "Parallel resistance (p.u.)"; C "Capacitance (p.u.)"
      mask init:
      | iC = 1./C;
      | iR = 1./R;
      | vssBlk = gcb;
      | switch dynamic
      |     case "Dynamic"
      |         set_param(vssBlk, 'LabelModeActiveChoice', 'dynamic');
      |     case "Static"
      |         set_param(vssBlk, 'LabelModeActiveChoice', 'static');
      |     case "Static omega"
      |         set_param(vssBlk, 'LabelModeActiveChoice', 'static omega');
      | end
      mask TypeOptions dynamic: Dynamic | Static | Static omega
  RL : Subsystem  Variant=on  VariantControlMode=label  LabelModeActiveChoice=dynamic  mask(Line){dynamic=Dynamic, R=Rf, L=Lf}
      mask prompts: dynamic "Dynamic behavior"; R "Series resistance (p.u.)"; L "Inductance (p.u.)"
      mask init:
      | invL = 1./L;
      | vssBlk = gcb;
      | switch dynamic
      |     case "Static"
      |         set_param(vssBlk, 'LabelModeActiveChoice', 'static');
      |     case "Dynamic"
      |         set_param(vssBlk, 'LabelModeActiveChoice', 'dynamic');
      |     case "Static omega"
      |         set_param(vssBlk, 'LabelModeActiveChoice', 'static_omega');
      | end
      mask Help: web('Documentation/RL.html')
      mask TypeOptions dynamic: Static | Dynamic | Static omega
  Real-Imag to Complex{2..5} (4 alike) : RealImagToComplex
  Relational Operator : RelationalOperator  Operator===  OutDataTypeStr=boolean  RndMeth=Simplest  InputSameDT=off
  Saturation : Saturate  UpperLimit=0.1  LowerLimit=0
  Scope{1,3,6..8} (5 alike) : Scope
      Scope1 settings: ActiveDisplayYMinimum=-0.06728  ActiveDisplayYMaximum=0.79818  DataLoggingVariableName=ScopeData2
      Scope3 settings: ActiveDisplayYMinimum=0.01769  ActiveDisplayYMaximum=0.10915
      Scope6 settings: ActiveDisplayYMinimum=0.03196  ActiveDisplayYMaximum=0.13112  DataLoggingVariableName=ScopeData2
      Scope7 settings: ActiveDisplayYMinimum=0.86043  ActiveDisplayYMaximum=1.1554  DataLoggingVariableName=ScopeData3
      Scope8 settings: ActiveDisplayYMinimum=0.0318  ActiveDisplayYMaximum=0.12782  DataLoggingVariableName=ScopeData4
  Scope2 : Scope  NumInputPorts=2
      settings: ActiveDisplayYMinimum=-0.10019  ActiveDisplayYMaximum=0.20176
  Scope4 : Scope  NumInputPorts=2
      settings: ActiveDisplayYMinimum=-0.04364  ActiveDisplayYMaximum=0.0791  DataLoggingVariableName=ScopeData3
  Sum1 : Sum  Inputs=++|
  Sum{3,5..6,9,14..15} (6 alike) : Sum  Inputs=|++
  Sum2 : Sum  Inputs=-+|
  Sum4 : Sum  Inputs=++|
  Sum8 : Sum  Inputs=-+|
  VI : Subsystem  mask{L=0.5, R=0.1, Tf=0}
      mask prompts: L "Inductance (pu)"; R "Resistance (pu)"; Tf "WOF time constant (s)"
      mask init: same as DCAC_conv_intconv_VSM/intconv_VSM/VI
  vidref : Outport
  viqref : Outport  Port=2
  wires:
  Product5/1 -> VI/2(iq)
  Product4/1 -> VI/1(id)
  Memory/1 -> Product4/1, Product5/1
  VI/2(vq) -> Sum15/2
  VI/1(vd) -> Sum14/1
  NOT/1 -> Memory/1
  voqref/1 -> Sum15/1  "voqref"
  vodref/1 -> Sum14/2  "vodref"
  Complex to Magnitude-Angle5/1 -> Scope8/1  "io_mod"
  Real-Imag to Complex5/1 -> Complex to Magnitude-Angle5/1
  Real-Imag to Complex4/1 -> Complex to Magnitude-Angle4/1
  Complex to Magnitude-Angle4/1 -> Scope7/1  "vc_mod"
  Complex to Magnitude-Angle3/2 -> Magnitude-Angle to Complex/2
  Magnitude-Angle to Complex/1 -> Complex to Real-Imag1/1
  Complex to Magnitude-Angle3/1 -> Saturation/1, Relational Operator/2, Scope6/1
  Relational Operator/1 -> NOT/1, PIvq/3(anti_windup), PIvd/3(anti_windup)
  Saturation/1 -> Relational Operator/1, Scope3/1, Magnitude-Angle to Complex/1
  Real-Imag to Complex3/1 -> Complex to Magnitude-Angle3/1
  Complex to Real-Imag1/1 -> PIid/1(ref), Scope2/2
  Complex to Magnitude-Angle2/1 -> Scope1/1  "i_mod"
  Real-Imag to Complex2/1 -> Complex to Magnitude-Angle2/1
  Complex to Real-Imag1/2 -> PIiq/1(ref), Scope4/2
  RC/1(vd) -> Cf 1/1, PIvd/2(y), vidref/1, [vod], Sum1/1, RL/2(v_out_d), Real-Imag to Complex4/1
  Sum5/1 -> [ilqref], Real-Imag to Complex3/2  "ilqref"
  Sum4/1 -> [ildref], Real-Imag to Complex3/1  "ildref"
  Sum6/1 -> RL/3(v_in_q)
  Sum1/1 -> RL/1(v_in_d)
  Sum9/1 -> Sum6/1  "viqref"
  Sum8/1 -> Sum1/2  "vidref"
  RL/2(iq) -> RC/3(i_q_in), Real-Imag to Complex2/2, "Lf "/1, PIiq/2(y), Scope4/1
  RL/1(id) -> Lf1/1, PIid/2(y), Real-Imag to Complex2/1, Scope2/1, RC/1(i_d_in)
  [omega] -> Product1/1
  omega/1 -> [omega], Product2/1  "omega"
  PIiq/1(Out1) -> Sum9/1
  PIid/1(Out1) -> Sum8/2
  PIvq/1(Out1) -> Sum3/1
  PIvd/1(Out1) -> Sum2/2
  Fi2/1 -> Sum5/2
  ioq/1 -> Product5/2, Real-Imag to Complex5/2, Fi2/1, RC/4(i_q_out)  "ioq"
  [omega] -> Product3/1, RL/5(omega), RC/5(omega)  "omega"
  Sum3/1 -> Sum5/1
  "Lf "/1 -> Product/1
  Sum2/1 -> Sum4/2
  iod/1 -> Fi/1, Product4/2, Real-Imag to Complex5/1, RC/2(i_d_out)  "iod"
  Product1/1 -> Sum2/1
  Cf/1 -> Product1/2
  Cf 1/1 -> Product2/2
  Product2/1 -> Sum3/2
  Product3/1 -> Sum9/2
  Sum15/1 -> PIvq/1(ref)  "voqref"
  Fi/1 -> Sum4/1
  Lf1/1 -> Product3/2
  [omega] -> Product/2
  RC/2(vq) -> Real-Imag to Complex4/2, Cf/1, PIvq/2(y), Sum6/2, RL/4(v_out_q), viqref/1, [voq]  "voq"
  Sum14/1 -> PIvd/1(ref)  "vodref"
  Product/1 -> Sum8/1

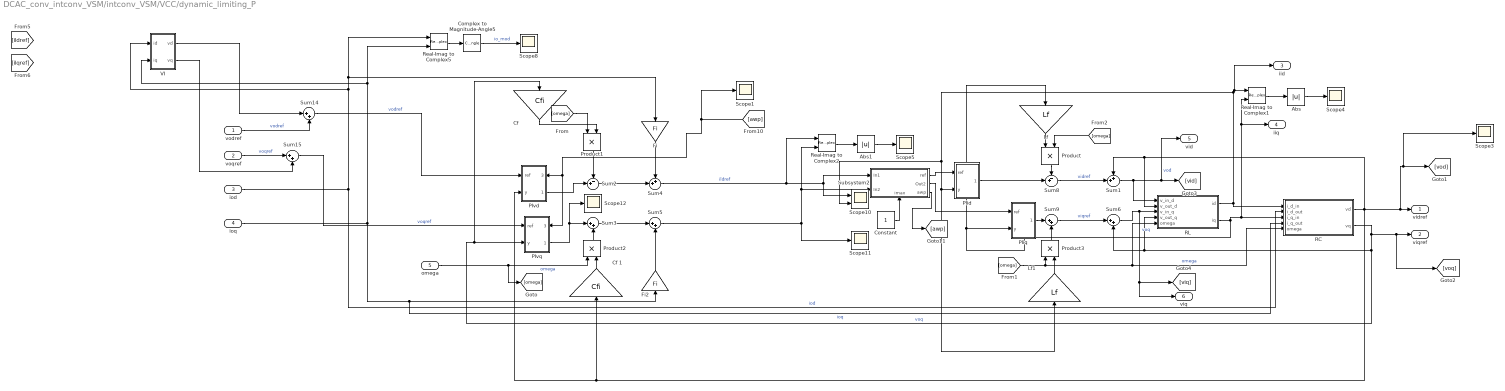
== system DCAC_conv_intconv_VSM/intconv_VSM/VCC/dynamic_limiting_P ==
  vodref : Inport
  voqref : Inport  Port=2
  iod : Inport  Port=3
  ioq : Inport  Port=4
  omega : Inport  Port=5
  Abs : Abs  SaturateOnIntegerOverflow=off
  Abs1 : Abs  SaturateOnIntegerOverflow=off
  Cf : Gain  Gain=Cfi
  Cf 1 : Gain  Gain=Cfi
  Complex to Magnitude-Angle5 : ComplexToMagnitudeAngle  Output=Magnitude
  Constant : Constant
  Fi : Gain  Gain=Fi
  Fi2 : Gain  Gain=Fi
  "Lf " : Gain  Gain=Lf
  Lf1 : Gain  Gain=Lf
  PIid : Subsystem
  PIiq : Subsystem
  PIvd : Subsystem
      settings: PortSchema="{\"entries\":[{\"content\":{\"sides\":[{\"content\":{\"connectorIds\":[\"In1\",\"In2\"]},\"type\":\"ConnectorPlacement.EquallySpacedRectSide\",\"uuid\":\"218efe14-094c-4cdd-8e62-ef6089c75bbd\"},{\"content\":{\"connectorIds\":[\"In3\",\"Out1\"],\"side\":\"RIGHT\"},\"type\":\"ConnectorPlacement.EquallySpacedRectSide\",\"uuid\":\"287e2a8a-062a-4519-a86c-f141c6982dac\"},{\"content\":{\"side\":\"TOP\"},\"type\":\"ConnectorPlacement.EquallySpacedRectSide\",\"uuid\":\"e88fce21-908c-492a-b265-04b05ce94be8\"}]},\"type\":\"ConnectorPlacement.EquallySpacedConnector\",\"uuid\":\"5c149457-da6d-4223-b1cb-56365173b759\"}],\"packageUris\":[\"http://schema.mathworks.com/mf0/Connector/R2020b\"],\"version\":\"1.0\"}"
  PIvq : Subsystem
      settings: PortSchema="{\"entries\":[{\"content\":{\"sides\":[{\"content\":{\"connectorIds\":[\"In1\",\"In2\"]},\"type\":\"ConnectorPlacement.EquallySpacedRectSide\",\"uuid\":\"5bfd4306-8421-4fdd-bae9-79740558d514\"},{\"content\":{\"connectorIds\":[\"In3\",\"Out1\"],\"side\":\"RIGHT\"},\"type\":\"ConnectorPlacement.EquallySpacedRectSide\",\"uuid\":\"1419fa8e-cc02-4da2-9592-d06db5fac946\"},{\"content\":{\"side\":\"TOP\"},\"type\":\"ConnectorPlacement.EquallySpacedRectSide\",\"uuid\":\"32aa87b6-be70-473d-807b-ed4692b27e5a\"}]},\"type\":\"ConnectorPlacement.EquallySpacedConnector\",\"uuid\":\"6bf6a9bf-c4c4-4ccc-a31e-1b4c70dd37d4\"}],\"packageUris\":[\"http://schema.mathworks.com/mf0/Connector/R2020b\"],\"version\":\"1.0\"}"
  Product{,1..3} (4 alike) : Product
  RC : Subsystem  Variant=on  VariantControlMode=label  LabelModeActiveChoice=dynamic  mask{dynamic=Dynamic, R=Rcf, C=Cfi}
      mask prompts: dynamic "Dynamic behavior"; R "Parallel resistance (p.u.)"; C "Capacitance (p.u.)"
      mask init: same as DCAC_conv_intconv_VSM/intconv_VSM/VCC/dynamic_limiting/RC
      mask TypeOptions dynamic: Dynamic | Static | Static omega
  RL : Subsystem  Variant=on  VariantControlMode=label  LabelModeActiveChoice=dynamic  mask(Line){dynamic=Dynamic, R=Rf, L=Lf}
      mask prompts: dynamic "Dynamic behavior"; R "Series resistance (p.u.)"; L "Inductance (p.u.)"
      mask init: same as DCAC_conv_intconv_VSM/intconv_VSM/VCC/dynamic_limiting/RL
      mask Help: web('Documentation/RL.html')
      mask TypeOptions dynamic: Static | Dynamic | Static omega
  Real-Imag to Complex1 : RealImagToComplex
  Real-Imag to Complex2 : RealImagToComplex
  Real-Imag to Complex5 : RealImagToComplex
  Scope{1,3..5,8,11..12} (7 alike) : Scope
      Scope1 settings: ActiveDisplayYMinimum=-0.125  ActiveDisplayYMaximum=1.125  DataLoggingVariableName=ScopeData2
      Scope11 settings: ActiveDisplayYMinimum=-166.4137  ActiveDisplayYMaximum=84.6213  DataLoggingVariableName=ScopeData2
      Scope12 settings: ActiveDisplayYMinimum=-1  ActiveDisplayYMaximum=1  DataLoggingVariableName=ScopeData3
      Scope3 settings: ActiveDisplayYMinimum=0.77192  ActiveDisplayYMaximum=1.1413  DataLoggingVariableName=ScopeData4
      Scope4 settings: ActiveDisplayYMinimum=0.18699  ActiveDisplayYMaximum=0.31058  DataLoggingVariableName=ScopeData6
      Scope5 settings: ActiveDisplayYMinimum=-1  ActiveDisplayYMaximum=1
      Scope8 settings: ActiveDisplayYMinimum=-1  ActiveDisplayYMaximum=1  DataLoggingVariableName=ScopeData4
  Scope10 : Scope  NumInputPorts=2
      settings: ActiveDisplayYMinimum=0.12846  ActiveDisplayYMaximum=0.33105
  Subsystem2 : Subsystem
      settings: PortSchema="{\"entries\":[{\"content\":{\"sides\":[{\"content\":{\"connectorIds\":[\"In1\",\"In2\"]},\"type\":\"ConnectorPlacement.EquallySpacedRectSide\",\"uuid\":\"9ad25d09-f130-47a3-8a0c-c3d50f40a3f5\"},{\"content\":{\"connectorIds\":[\"Out1\",\"Out2\",\"Out3\"],\"side\":\"RIGHT\"},\"type\":\"ConnectorPlacement.EquallySpacedRectSide\",\"uuid\":\"00c4c943-52e8-4170-9ba5-4d3b10561d7b\"},{\"content\":{\"side\":\"TOP\"},\"type\":\"ConnectorPlacement.EquallySpacedRectSide\",\"uuid\":\"98a959d8-b430-483b-8e6f-0eab01c1bae1\"},{\"content\":{\"connectorIds\":[\"In3\"],\"side\":\"BOTTOM\"},\"type\":\"ConnectorPlacement.EquallySpacedRectSide\",\"uuid\":\"01418333-d465-4764-adcc-2e5b92b6bf5d\"}]},\"type\":\"ConnectorPlacement.EquallySpacedConnector\",\"uuid\":\"e741d9d4-93b5-4bd9-8695-3e699c12860d\"}],\"packageUris\":[\"http://schema.mathworks.com/mf0/Connector/R2020b\"],\"version\":\"1.0\"}"
  Sum1 : Sum  Inputs=++|
  Sum{3,5..6,9,14..15} (6 alike) : Sum  Inputs=|++
  Sum2 : Sum  Inputs=-+|
  Sum4 : Sum  Inputs=++|
  Sum8 : Sum  Inputs=-+|
  VI : Subsystem  mask{L=0, R=0, Tf=0}
      mask prompts: L "Inductance (pu)"; R "Resistance (pu)"; Tf "WOF time constant (s)"
      mask init: same as DCAC_conv_intconv_VSM/intconv_VSM/VI
  vidref : Outport
  viqref : Outport  Port=2
  iid : Outport  Port=3
  iiq : Outport  Port=4
  vid : Outport  Port=5
  viq : Outport  Port=6
  wires:
  Sum4/1 -> Scope10/1, Subsystem2/1(In1), Real-Imag to Complex2/1  "ildref"
  Subsystem2/3(awp) -> [awp]
  Constant/1 -> Subsystem2/3(imax)
  Subsystem2/2(Out2) -> PIiq/1(ref)
  Subsystem2/1(ref) -> PIid/1(ref)
  Fi2/1 -> Sum5/2
  Product2/1 -> Sum3/2
  [awp] -> Scope1/1, PIvq/3(awp), PIvd/3(awp)
  Fi/1 -> Sum4/1
  Abs1/1 -> Scope5/1
  Real-Imag to Complex2/1 -> Abs1/1
  Sum5/1 -> Scope11/1, Real-Imag to Complex2/2, Subsystem2/2(In2)
  Real-Imag to Complex1/1 -> Abs/1
  Abs/1 -> Scope4/1
  Sum1/1 -> [vid], vid/1, RL/1(v_in_d)  "vod"
  Sum6/1 -> RL/3(v_in_q), [viq], viq/1  "voq"
  VI/2(vq) -> Sum15/2
  VI/1(vd) -> Sum14/1
  voqref/1 -> Sum15/1  "voqref"
  vodref/1 -> Sum14/2  "vodref"
  Complex to Magnitude-Angle5/1 -> Scope8/1  "io_mod"
  Real-Imag to Complex5/1 -> Complex to Magnitude-Angle5/1
  RC/1(vd) -> Cf 1/1, PIvd/2(y), vidref/1, [vod], Scope3/1, Sum1/1, RL/2(v_out_d)
  Sum9/1 -> Sum6/1  "viqref"
  Sum8/1 -> Sum1/2  "vidref"
  RL/2(iq) -> RC/3(i_q_in), Real-Imag to Complex1/2, iiq/1, "Lf "/1, PIiq/2(y)
  RL/1(id) -> Scope10/2, Lf1/1, PIid/2(y), Real-Imag to Complex1/1, iid/1, RC/1(i_d_in)
  [omega] -> Product1/1
  omega/1 -> Product2/1, [omega]  "omega"
  PIiq/1(Out1) -> Sum9/1
  PIid/1(Out1) -> Sum8/2
  PIvq/1(Out1) -> Sum3/1, Scope12/1
  PIvd/1(Out1) -> Sum2/2
  ioq/1 -> Real-Imag to Complex5/2, VI/2(iq), Fi2/1, RC/4(i_q_out)  "ioq"
  [omega] -> Product3/1, RC/5(omega), RL/5(omega)  "omega"
  Sum3/1 -> Sum5/1
  "Lf "/1 -> Product/1
  Sum2/1 -> Sum4/2
  iod/1 -> RC/2(i_d_out), Real-Imag to Complex5/1, Fi/1, VI/1(id)  "iod"
  Product1/1 -> Sum2/1
  Cf/1 -> Product1/2
  Cf 1/1 -> Product2/2
  Product3/1 -> Sum9/2
  Sum15/1 -> PIvq/1(ref)  "voqref"
  Lf1/1 -> Product3/2
  [omega] -> Product/2
  RC/2(vq) -> Cf/1, PIvq/2(y), Sum6/2, RL/4(v_out_q), viqref/1, [voq]  "voq"
  Sum14/1 -> PIvd/1(ref)  "vodref"
  Product/1 -> Sum8/1

== system DCAC_conv_intconv_VSM/intconv_VSM/VCC/static ==
  vodref : Inport
  voqref : Inport  Port=2
  iod : Inport  Port=3
  ioq : Inport  Port=4
  omega : Inport  Port=5
  Terminator : Terminator
  Terminator1 : Terminator
  Terminator2 : Terminator
  vidref : Outport
  viqref : Outport  Port=2
  wires:
  omega/1 -> Terminator2/1  "ioq"
  ioq/1 -> Terminator1/1  "ioq"
  iod/1 -> Terminator/1  "iod"
  vodref/1 -> vidref/1  "vodref"
  voqref/1 -> viqref/1  "voqref"

== system DCAC_conv_intconv_VSM/intconv_VSM/VI/WOF_d ==
  In1 : Inport
  Gain : Gain  Gain=iTf
  I : Integrator  InitialConditionSource=external  InitialCondition=Grid_op_VCVSC.op.States(6).x'
  Sum : Sum  Inputs=+-|
  Sum4 : Sum  Inputs=|+-
  Out1 : Outport
  wires:
  Gain/1 -> I/1
  Sum4/1 -> Gain/1
  In1/1 -> I/2, Sum/1, Sum4/1
  I/1 -> Sum/2, Sum4/2
  Sum/1 -> Out1/1

== system DCAC_conv_intconv_VSM/intconv_VSM/VI/WOF_q ==
  In1 : Inport
  Gain : Gain  Gain=iTf
  I : Integrator  InitialConditionSource=external  InitialCondition=Grid_op_VCVSC.op.States(7).x'
  Sum : Sum  Inputs=+-|
  Sum4 : Sum  Inputs=|+-
  Out1 : Outport
  wires:
  Gain/1 -> I/1
  Sum4/1 -> Gain/1
  In1/1 -> I/2, Sum/1, Sum4/1
  I/1 -> Sum/2, Sum4/2
  Sum/1 -> Out1/1

== system DCAC_conv_intconv_VSM/intconv_VSM/VCC/dynamic/PIid ==
  ref : Inport
  y : Inport  Port=2
  Gain : Gain  Gain=Bint
  Gain1 : Gain  Gain=1/Tint
  Gain2 : Gain  Gain=Kint
  I : Integrator  InitialCondition=Grid_opintconv_VSM.PIid
  Sum : Sum  Inputs=++|
  Sum1 : Sum  Inputs=|+-
  Sum6 : Sum  Inputs=|+-
  Out1 : Outport
  wires:
  Gain2/1 -> Out1/1
  I/1 -> Sum/2
  Gain1/1 -> I/1
  Sum6/1 -> Gain1/1
  Sum1/1 -> Sum/1
  Sum/1 -> Gain2/1
  Gain/1 -> Sum1/1
  ref/1 -> Sum6/1, Gain/1
  y/1 -> Sum6/2, Sum1/2
